simulink model "Cell_model"  (R2023a)
settings: Solver=VariableStepAuto  StartTime=0.0  StopTime=10.0  RelTol=1e-3
libraries: simulink x2
settings Model: Creator=Lenovo  LastModifiedBy=Lenovo

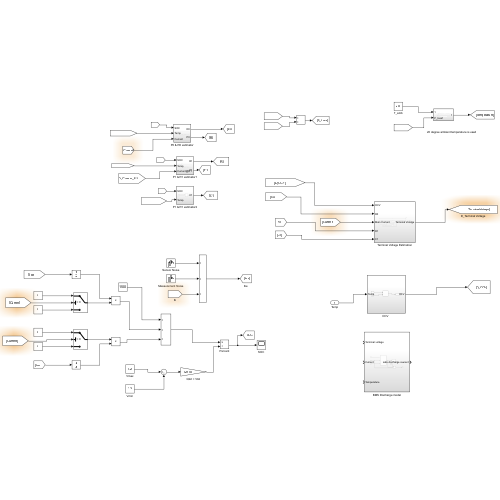
[thumbnail: Simulink's stored preview of the top-level diagram]
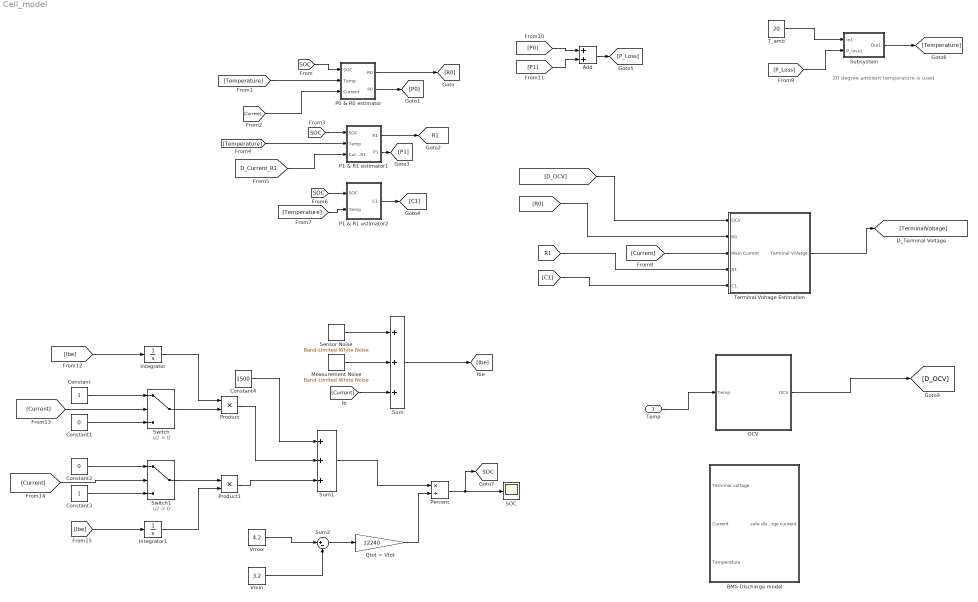
== system Cell_model ==
  note: 20 degree ambient temperature is used
  Temp : Inport
  Add : Sum
  BMS Discharge model : Subsystem
  Constant : Constant
  Constant1 : Constant  Value=0
  Constant2 : Constant  Value=0
  Constant3 : Constant
  Constant4 : Constant  Value=1500
  Integrator : Integrator
  Integrator1 : Integrator
  Measurement Noise : simulink/Sources/Band-Limited White Noise  Cov=[0.1]  Ts=0.1  seed=[23341]
  "OCV  " : Subsystem
  P0 & R0 estimator : Subsystem
  P1 & R1 estimator1 : Subsystem
  P1 & R1 estimator2 : Subsystem
  Percent : Product  Inputs=*/
  Product : Product
  Product1 : Product
  Qtot = Vtot : Gain  Gain=12240
  SOC : Scope
  Sensor Noise : simulink/Sources/Band-Limited White Noise  Cov=[0.1]  Ts=0.1  seed=[23341]
  Subsystem : Subsystem
  Sum : Sum  Inputs=+++
  Sum1 : Sum  Inputs=+++
  Sum2 : Sum  Inputs=|+-
  Switch : Switch  Criteria=u2 > Threshold  SaturateOnIntegerOverflow=off  InputSameDT=off
  Switch1 : Switch  Criteria=u2 > Threshold  SaturateOnIntegerOverflow=off  InputSameDT=off
  T_amb : Constant  Value=20
  Terminal Voltage Estimation : Subsystem
  Vmax : Constant  Value=4.2
  Vmin : Constant  Value=3.2
  tag scope: R1=global, SOC=global
  wires:
  [SOC] -> P0 & R0 estimator/1(SOC)
  [Temperature] -> P0 & R0 estimator/2(Temp)
  [Current] -> P0 & R0 estimator/3(Current)
  P0 & R0 estimator/1(R0) -> [R0]
  P0 & R0 estimator/2(P0) -> [P0]
  [D_Current_R1] -> P1 & R1 estimator1/3(Current@R1)
  P1 & R1 estimator1/2(P1) -> [P1]
  [Temperature] -> P1 & R1 estimator1/2(Temp)
  [SOC] -> P1 & R1 estimator1/1(SOC)
  P1 & R1 estimator1/1(R1) -> [R1]
  [Temperature] -> P1 & R1 estimator2/2(Temp)
  [SOC] -> P1 & R1 estimator2/1(SOC)
  P1 & R1 estimator2/1(C1) -> [C1]
  Add/1 -> [P_Loss]
  [D_OCV] -> Terminal Voltage Estimation/1(OCV)
  [C1] -> Terminal Voltage Estimation/5(C1)
  [R1] -> Terminal Voltage Estimation/4(R1)
  Terminal Voltage Estimation/1(Terminal Volatge) -> [TerminalVoltage]
  [R0] -> Terminal Voltage Estimation/2(R0)
  T_amb/1 -> Subsystem/1(In1)
  Subsystem/1(Out1) -> [Temperature]
  [Current] -> Terminal Voltage Estimation/3(Main Current)
  [P_Loss] -> Subsystem/2(P_loss1)
  [P1] -> Add/2
  [P0] -> Add/1
  Sensor Noise/1 -> Sum/1
  Vmin/1 -> Sum2/2
  Integrator/1 -> Product/1
  Sum2/1 -> Qtot = Vtot/1
  [Current] -> Switch1/2
  Constant/1 -> Switch/1
  Product/1 -> Sum1/2
  Switch/1 -> Product/2
  Vmax/1 -> Sum2/1
  Constant4/1 -> Sum1/1
  Switch1/1 -> Product1/1
  Qtot = Vtot/1 -> Percent/2
  [Ibe] -> Integrator1/1
  Sum/1 -> [Ibe]
  Sum1/1 -> Percent/1
  Constant3/1 -> Switch1/3
  Measurement Noise/1 -> Sum/2
  Percent/1 -> [SOC], SOC/1
  Constant1/1 -> Switch/3
  Integrator1/1 -> Product1/2
  [Ibe] -> Integrator/1
  [Current] -> Sum/3
  [Current] -> Switch/2
  Constant2/1 -> Switch1/1
  Product1/1 -> Sum1/3
  Temp/1 -> "OCV  "/1(Temp)
  "OCV  "/1(OCV) -> [D_OCV]

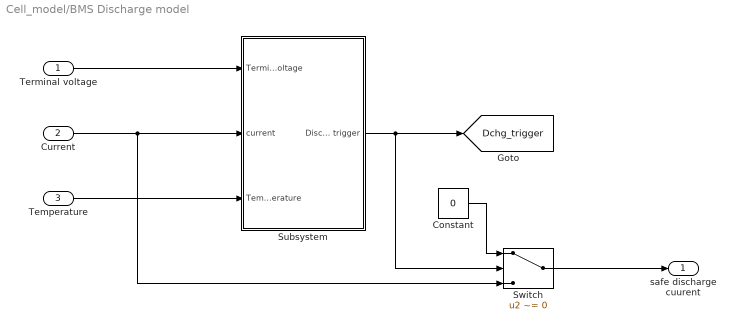
== system Cell_model/BMS Discharge model ==
  Terminal voltage : Inport
  Current : Inport  Port=2
  Temperature : Inport  Port=3
  Constant : Constant  Value=0
  Subsystem : Subsystem
  Switch : Switch  Criteria=u2 ~= 0  SaturateOnIntegerOverflow=off  InputSameDT=off
  safe discharge cuurent : Outport
  tag scope: Dchg_trigger=global
  wires:
  Terminal voltage/1 -> Subsystem/1(Terminal Voltage)
  Current/1 -> Switch/3, Subsystem/2(current)
  Temperature/1 -> Subsystem/3(Temperature)
  Subsystem/1(Discharge trigger) -> Switch/2, [Dchg_trigger]
  Constant/1 -> Switch/1
  Switch/1 -> safe discharge cuurent/1

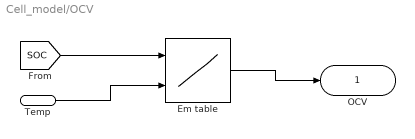
== system Cell_model/OCV   ==
  Temp : Inport
  Em table : Lookup_n-D  BreakpointsForDimension1=[1:3]  BreakpointsForDimension2=[1:3]  InternalRulePriority=Speed  RndMeth=Simplest
      settings: InputPortMap=u0,u1
  OCV : Outport
  wires:
  Temp/1 -> Em table/2
  Em table/1 -> OCV/1
  [SOC] -> Em table/1

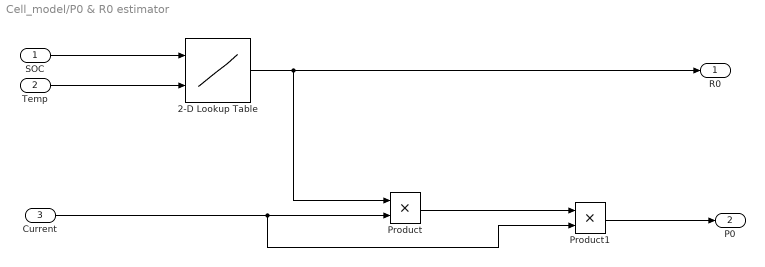
== system Cell_model/P0 & R0 estimator ==
  SOC : Inport
  Temp : Inport  Port=2
  Current : Inport  Port=3
  2-D Lookup Table : Lookup_n-D  BreakpointsForDimension1=[1:3]  BreakpointsForDimension2=[1:3]  InternalRulePriority=Speed  RndMeth=Simplest
      settings: InputPortMap=u0,u1
  Product : Product
  Product1 : Product
  R0 : Outport
  P0 : Outport  Port=2
  wires:
  Product1/1 -> P0/1
  SOC/1 -> 2-D Lookup Table/1
  Current/1 -> Product1/2, Product/2
  2-D Lookup Table/1 -> R0/1, Product/1
  Temp/1 -> 2-D Lookup Table/2
  Product/1 -> Product1/1

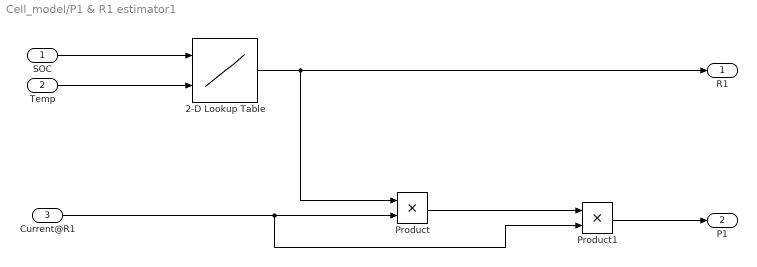
== system Cell_model/P1 & R1 estimator1 ==
  SOC : Inport
  Temp : Inport  Port=2
  Current@R1 : Inport  Port=3
  2-D Lookup Table : Lookup_n-D  BreakpointsForDimension1=[1:3]  BreakpointsForDimension2=[1:3]  InternalRulePriority=Speed  RndMeth=Simplest
      settings: InputPortMap=u0,u1
  Product : Product
  Product1 : Product
  R1 : Outport
  P1 : Outport  Port=2
  wires:
  Product1/1 -> P1/1
  SOC/1 -> 2-D Lookup Table/1
  Current@R1/1 -> Product1/2, Product/2
  2-D Lookup Table/1 -> R1/1, Product/1
  Temp/1 -> 2-D Lookup Table/2
  Product/1 -> Product1/1

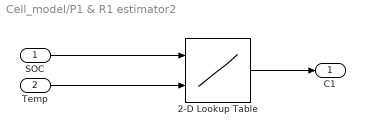
== system Cell_model/P1 & R1 estimator2 ==
  SOC : Inport
  Temp : Inport  Port=2
  2-D Lookup Table : Lookup_n-D  BreakpointsForDimension1=[1:3]  BreakpointsForDimension2=[1:3]  InternalRulePriority=Speed  RndMeth=Simplest
      settings: InputPortMap=u0,u1
  C1 : Outport
  wires:
  SOC/1 -> 2-D Lookup Table/1
  2-D Lookup Table/1 -> C1/1
  Temp/1 -> 2-D Lookup Table/2

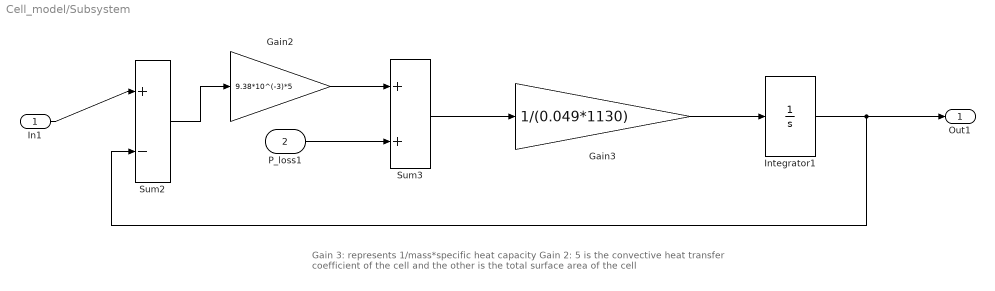
== system Cell_model/Subsystem ==
  note: Gain 3: represents 1/mass*specific heat capacity
      | Gain 2: 5 is the convective heat transfer coefficient of the cell and the other is the total surface area of the cell
  In1 : Inport
  P_loss1 : Inport  Port=2
  Gain2 : Gain  Gain=9.38*10^(-3)*5
  Gain3 : Gain  Gain=1/(0.049*1130)
  Integrator1 : Integrator
  Sum2 : Sum  Inputs=|+-
  Sum3 : Sum
  Out1 : Outport
  wires:
  In1/1 -> Sum2/1
  Sum3/1 -> Gain3/1
  Sum2/1 -> Gain2/1
  P_loss1/1 -> Sum3/2
  Gain3/1 -> Integrator1/1
  Integrator1/1 -> Out1/1, Sum2/2
  Gain2/1 -> Sum3/1

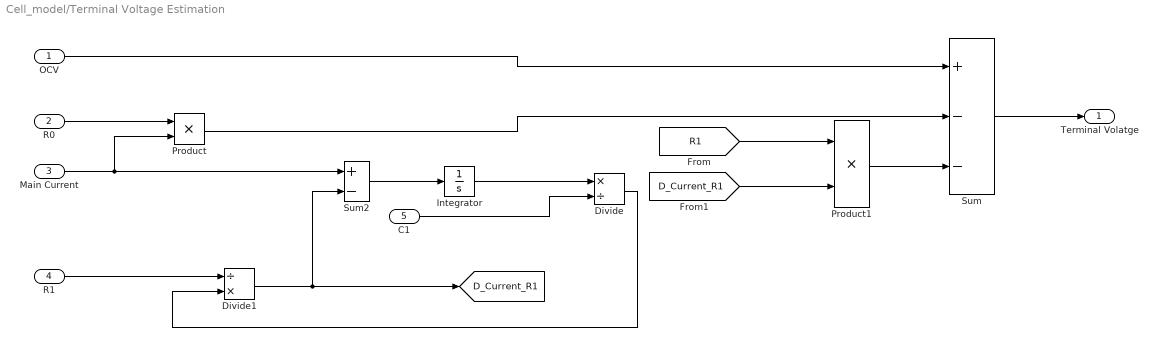
== system Cell_model/Terminal Voltage Estimation ==
  OCV : Inport
  R0 : Inport  Port=2
  Main Current : Inport  Port=3
  R1 : Inport  Port=4
  C1 : Inport  Port=5
  Divide : Product  Inputs=*/
  Divide1 : Product  Inputs=/*
  Integrator : Integrator
  Product : Product
  Product1 : Product
  Sum : Sum  Inputs=+--
  Sum2 : Sum  Inputs=+-
  Terminal Volatge : Outport
  tag scope: D_Current_R1=global
  wires:
  [D_Current_R1] -> Product1/2
  R0/1 -> Product/1
  Product/1 -> Sum/2
  Sum/1 -> Terminal Volatge/1
  Product1/1 -> Sum/3
  Divide/1 -> Divide1/2
  C1/1 -> Divide/2
  Integrator/1 -> Divide/1
  Sum2/1 -> Integrator/1
  Main Current/1 -> Sum2/1, Product/2
  [R1] -> Product1/1
  Divide1/1 -> [D_Current_R1], Sum2/2
  OCV/1 -> Sum/1
  R1/1 -> Divide1/1

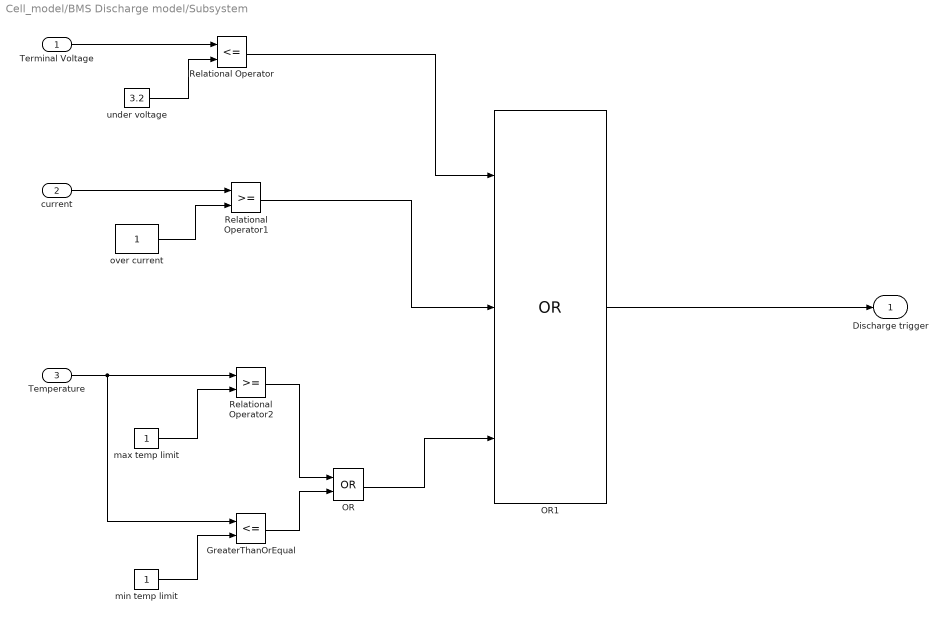
== system Cell_model/BMS Discharge model/Subsystem ==
  Terminal Voltage : Inport
  current : Inport  Port=2
  Temperature : Inport  Port=3
  GreaterThanOrEqual : RelationalOperator  Operator=<=  OutDataTypeStr=boolean  RndMeth=Simplest  InputSameDT=off
  OR : Logic  Operator=OR  AllPortsSameDT=off  OutDataTypeStr=boolean
  OR1 : Logic  Operator=OR  Inputs=3  AllPortsSameDT=off  OutDataTypeStr=boolean
  Relational Operator : RelationalOperator  Operator=<=  OutDataTypeStr=boolean  RndMeth=Simplest  InputSameDT=off
  Relational Operator1 : RelationalOperator  OutDataTypeStr=boolean  RndMeth=Simplest  InputSameDT=off
  Relational Operator2 : RelationalOperator  OutDataTypeStr=boolean  RndMeth=Simplest  InputSameDT=off
  max temp limit : Constant
  min temp limit : Constant
  over current : Constant
  under voltage : Constant  Value=3.2
  Discharge trigger : Outport
  wires:
  Terminal Voltage/1 -> Relational Operator/1
  under voltage/1 -> Relational Operator/2
  current/1 -> Relational Operator1/1
  over current/1 -> Relational Operator1/2
  Temperature/1 -> GreaterThanOrEqual/1, Relational Operator2/1
  max temp limit/1 -> Relational Operator2/2
  min temp limit/1 -> GreaterThanOrEqual/2
  Relational Operator2/1 -> OR/1
  GreaterThanOrEqual/1 -> OR/2
  Relational Operator/1 -> OR1/1
  Relational Operator1/1 -> OR1/2
  OR/1 -> OR1/3
  OR1/1 -> Discharge trigger/1
